simulink model "Kal_pitch_sim"  (R2023b)
settings: Solver=FixedStepAuto  StartTime=0.0  StopTime=50  FixedStep=0.001  RelTol=1e-3
values from neighbouring files (symbols this model uses):
  beta = pi/10    (= 0.314159265359)    [Kal_6Dpitch_mat.m]    (also in Kal_pitch_mat.m; TestValori.m = 0.523598775598; TestVel.m = 0.523598775598)
  cov_ic = [10, 0 ... (first row only)    [KalPrep_mat.m]    (also in Kal_6Dpitch_mat.m = cov_ic * (1 + 2*rand); Kal_pitch_mat.m = cov_ic * (1 + 2*rand))
  eta1 = deg2rad(1)    [KalPrep_mat.m]    (also in Kal_6Dpitch_mat.m = 0.05; Kal_pitch_mat.m = 0.05)
  eta2 = 0.05    [Kal_6Dpitch_mat.m]    (also in Kal_pitch_mat.m)
  G = [Ts 0 ... (first row only)    [KalPrep_mat.m]    (also in Kal_6Dpitch_mat.m = eye(3) * Ts; Kal_pitch_mat.m = eye(3) * Ts)
  Gamma = -pi/6    (= -0.523598775598)    [Kal_6Dpitch_mat.m]    (also in Kal_pitch_mat.m; TestValori.m)
  init_cond = [pi/2; 5]    [KalPrep_mat.m]    (also in Kal_6Dpitch_mat.m = [2; 0; 0]; Kal_pitch_mat.m = [2; 0; 0])
  Lambda = pi/6    (= 0.523598775598)    [Kal_6Dpitch_mat.m]    (also in Kal_pitch_mat.m; TestValori.m)
  pr0 = [0,0]'    [Kal_6Dpitch_mat.m]    (also in Kal_pitch_mat.m)
  Q = [(sig1^2), 0 ... (first row only)    [KalPrep_mat.m]    (also in Kal_6Dpitch_mat.m = zeros(3,3); Kal_pitch_mat.m = zeros(3,3))
  qt = - 10    (= -10)    [Kal_6Dpitch_mat.m]    (also in Kal_pitch_mat.m; TestValori.m = -5)
  R = (eta1)^2    [KalPrep_mat.m]    (also in Kal_6Dpitch_mat.m = [(eta1^2), 0; Kal_pitch_mat.m = [(eta1^2), 0; untitled.m = 10)
  sig1 = 0.1    [KalPrep_mat.m]    (also in Kal_6Dpitch_mat.m; Kal_pitch_mat.m)
  sig2 = 0.2    [KalPrep_mat.m]    (also in Kal_6Dpitch_mat.m; Kal_pitch_mat.m)
  sig3 = 0.15    [Kal_6Dpitch_mat.m]    (also in Kal_pitch_mat.m)
  Ts = 0.001    [KalPrep_mat.m]    (also in Kal_6Dpitch_mat.m; Kal_pitch_mat.m; TestVel.m)
  v_heave = 0.00    (= 0)    [Kal_pitch_mat.m]
  v_surge = 0.5    [Kal_pitch_mat.m]
settings Model: Creator=fabio  LastModifiedBy=fabio

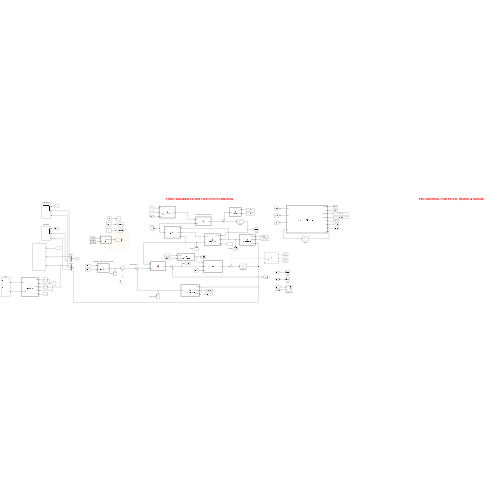
[thumbnail: Simulink's stored preview of the top-level diagram]
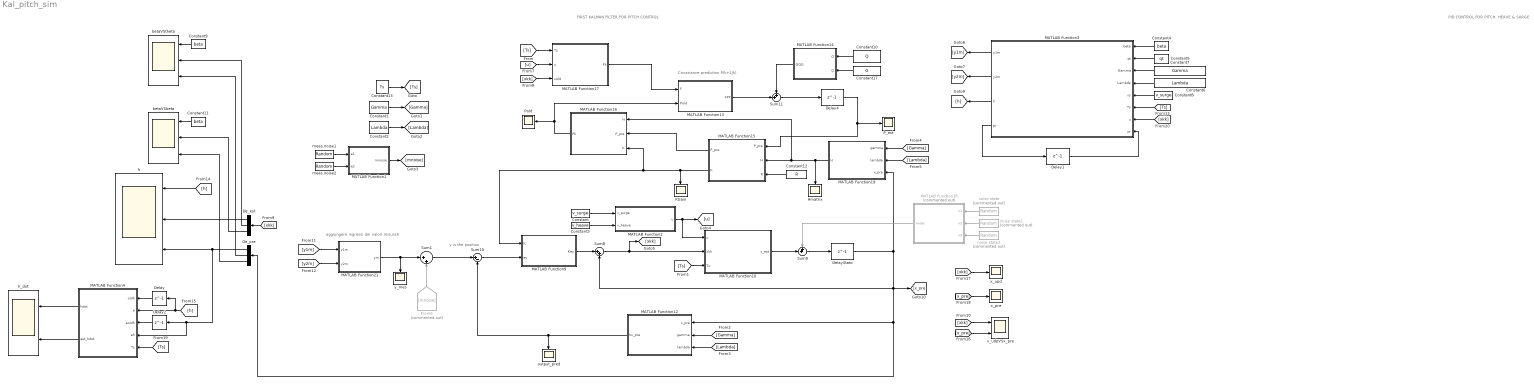
== system Kal_pitch_sim ==
  note: aggiungere ingressi dei valorì misurati
  note: Covariance prediction P(k+1|k)
  note: FIRST KALMAN FILTER FOR PITCH CONTROL
  note: y is the position
  note: PID CONTROL FOR PITCH, HEAVE & SURGE
  Constant : Constant  Value=v_surge
  Constant1 : Constant  Value=Gamma
  Constant10 : Constant  Value=Q  VectorParams1D=off
  Constant11 : Constant  Value=beta
  Constant12 : Constant  Value=R
  Constant13 : Constant  Value=Ts
  Constant17 : Constant  Value=G  VectorParams1D=off
  Constant2 : Constant  Value=Lambda
  Constant3 : Constant  Value=v_heave
  Constant4 : Constant  Value=beta
  Constant5 : Constant  Value=qt
  Constant6 : Constant  Value=Lambda
  Constant7 : Constant  Value=Gamma
  Constant8 : Constant  Value=v_surge
  Constant9 : Constant  Value=beta
  De_est : Demux  Outputs=3
  De_pre : Demux  Outputs=3
  Delay : Delay  DelayLength=1
  Delay1 : Delay  DelayLength=1  InitialCondition=pr0  UseCircularBuffer=on
  Delay2 : Delay  DelayLength=1
  Delay4 : Delay  DelayLength=1  InitialCondition=cov_ic  UseCircularBuffer=on
  DelayStato : Delay  DelayLength=1  InitialCondition=init_cond  UseCircularBuffer=on
  From6 : From  Commented=on  GotoTag=mnoise
  Hmatrix : Scope
  KGain : Scope
  MATLAB Function1 : MATLAB Function  TreatAsAtomicUnit=on
  MATLAB Function10 : MATLAB Function  TreatAsAtomicUnit=on
  MATLAB Function12 : MATLAB Function  TreatAsAtomicUnit=on
  MATLAB Function13 : MATLAB Function  TreatAsAtomicUnit=on
  MATLAB Function14 : MATLAB Function  TreatAsAtomicUnit=on
  MATLAB Function15 : MATLAB Function  TreatAsAtomicUnit=on
  MATLAB Function16 : MATLAB Function  TreatAsAtomicUnit=on
  MATLAB Function17 : MATLAB Function  TreatAsAtomicUnit=on
  MATLAB Function18 : MATLAB Function  Commented=on  TreatAsAtomicUnit=on
  MATLAB Function19 : MATLAB Function  TreatAsAtomicUnit=on
  MATLAB Function2 : MATLAB Function  TreatAsAtomicUnit=on
  MATLAB Function21 : MATLAB Function  TreatAsAtomicUnit=on
  MATLAB Function3 : MATLAB Function  TreatAsAtomicUnit=on
  MATLAB Function4 : MATLAB Function  TreatAsAtomicUnit=on
  MATLAB Function9 : MATLAB Function  TreatAsAtomicUnit=on
  P_est : Scope
  Pold : Scope
  Sum1 : Sum  Inputs=|++
  Sum10 : Sum  Inputs=|+-
  Sum11 : Sum  Inputs=++|
  Sum8 : Sum  Inputs=|++
  Sum9 : Sum  Inputs=++|
  betaVSbeta : Scope  NumInputPorts=3
  betaVStheta : Scope  NumInputPorts=3
  h : Scope  NumInputPorts=3
  h_dot : Scope  NumInputPorts=2
  meas.noise1 : RandomNumber  Variance=eta1  SampleTime=Ts
  meas.noise2 : RandomNumber  Variance=eta2  SampleTime=Ts
  noise state : RandomNumber  Commented=on  Variance=sig1  SampleTime=Ts
  noise state1 : RandomNumber  Commented=on  Variance=sig2  SampleTime=Ts
  noise state2 : RandomNumber  Commented=on  Variance=sig3  SampleTime=Ts
  output_pred : Scope
  x_pre : Scope
  x_udpVSx_pre : Scope  NumInputPorts=2
  x_upd : Scope
  y_mes : Scope
  wires:
  MATLAB Function17/1(Fk) -> MATLAB Function13/1(F)
  DelayStato/1 -> Sum8/2, [x_pre], MATLAB Function12/1(x_pre), De_pre/1, MATLAB Function19/3(x_pre)
  Delay4/1 -> P_est/1, MATLAB Function15/1("P_pre ")
  MATLAB Function12/1(hx_pre) -> Sum10/2, output_pred/1
  Sum10/1 -> MATLAB Function9/2(ey)
  MATLAB Function19/1(H) -> Hmatrix/1, MATLAB Function16/1(H), MATLAB Function15/2(H)
  Constant17/1 -> MATLAB Function14/2(G)
  MATLAB Function14/1(GQG) -> Sum11/1
  MATLAB Function13/1(FPF) -> Sum11/2
  Constant10/1 -> MATLAB Function14/1(Q)
  MATLAB Function10/1(x_est) -> Sum9/2
  MATLAB Function16/1(Pk) -> Pold/1, MATLAB Function13/2(Pold)
  Sum9/1 -> DelayStato/1
  Constant12/1 -> MATLAB Function15/3(R)
  MATLAB Function15/2(K) -> KGain/1, MATLAB Function16/3(K), MATLAB Function9/1(K)
  Sum11/1 -> Delay4/1
  Sum8/1 -> [xkk], MATLAB Function10/2(xkk)
  MATLAB Function15/1(P_pre) -> MATLAB Function16/2(P_pre)
  MATLAB Function9/1(Key) -> Sum8/1
  MATLAB Function21/1(ym) -> y_mes/1, Sum1/1
  Constant13/1 -> [Ts]
  [Ts] -> MATLAB Function17/1(Ts)
  [Ts] -> MATLAB Function10/3(Ts)
  Constant1/1 -> [Gamma]
  Constant2/1 -> [Lambda]
  [Gamma] -> MATLAB Function12/2(gamma)
  [Lambda] -> MATLAB Function12/3(lambda)
  [Gamma] -> MATLAB Function19/1(gamma)
  [Lambda] -> MATLAB Function19/2(lambda)
  noise state/1 -> MATLAB Function18/1(n1)
  noise state2/1 -> MATLAB Function18/3(n3)
  noise state1/1 -> MATLAB Function18/2(n2)
  MATLAB Function18/1(noise) -> Sum9/1
  Sum1/1 -> Sum10/1
  meas.noise1/1 -> MATLAB Function1/1(e1)
  meas.noise2/1 -> MATLAB Function1/2(e2)
  MATLAB Function1/1(mnoise) -> [mnoise]
  Constant/1 -> MATLAB Function2/1(v_surge)
  MATLAB Function2/1(u) -> MATLAB Function10/1(u), [u]
  [u] -> MATLAB Function17/2(u)
  [xkk] -> MATLAB Function17/3(xold)
  Delay1/1 -> MATLAB Function3/8("pr ")
  MATLAB Function3/4(pr) -> Delay1/1
  MATLAB Function3/1(y1m) -> [y1m]
  MATLAB Function3/2(y2m) -> [y2m]
  [y1m] -> MATLAB Function21/1(y1m)
  [y2m] -> MATLAB Function21/2(y2m)
  Constant4/1 -> MATLAB Function3/1(beta)
  Constant5/1 -> MATLAB Function3/2(qt)
  Constant6/1 -> MATLAB Function3/4(Lambda)
  Constant8/1 -> MATLAB Function3/5(vs)
  [Ts] -> MATLAB Function3/6(Ts)
  MATLAB Function3/3(h) -> [h]
  [h] -> h/1
  [xkk] -> De_est/1
  De_est/1 -> h/2
  De_pre/1 -> MATLAB Function4/4(eh), Delay2/1, h/3
  Constant9/1 -> betaVStheta/1
  Constant7/1 -> MATLAB Function3/3(Gamma)
  MATLAB Function4/1(hdot) -> h_dot/1
  De_est/2 -> betaVStheta/2
  De_pre/2 -> betaVStheta/3
  De_est/3 -> betaVSbeta/2
  De_pre/3 -> betaVSbeta/3
  Constant11/1 -> betaVSbeta/1
  Constant3/1 -> MATLAB Function2/2(v_heave)
  [xkk] -> x_udpVSx_pre/1
  [x_pre] -> x_udpVSx_pre/2
  [xkk] -> x_upd/1
  [x_pre] -> x_pre/1
  MATLAB Function4/2(est_hdot) -> h_dot/2
  [h] -> Delay/1, MATLAB Function4/2(h)
  Delay/1 -> MATLAB Function4/1(oldh)
  Delay2/1 -> MATLAB Function4/3(eoldh)
  [Ts] -> MATLAB Function4/5(Ts)
  [xkk] -> MATLAB Function3/7(x)
  From6/1 -> Sum1/2

== matlab function Kal_pitch_sim/MATLAB Function16 ==
  data: H input; P_pre input; Pk output; K input
function Pk = PkComp(H ,P_pre, K)
    s = size((K*H), 1);
    I = eye(s); 
    Pk = (I - K*H)*P_pre;

== matlab function Kal_pitch_sim/MATLAB Function9 ==
  data: K input; ey input; Key output
function Key = GainMult(K, ey)
    Key = K*ey;

== matlab function Kal_pitch_sim/MATLAB Function17 ==
  data: Fk output; Ts input; u input; xold input
function Fk = DynamicJacobian(Ts, u, xold)
    delta = xold(3) - xold(2);
    % u(1) = vsurge, u(2) = vheave
    % !! ATTENZIONE:
    % STO CONSIDERANDO H RISPETTO TERRAIN FRAME E THETA E BETA RISPETTO
    % INERZIALE
    F = [0, -u(1)*cos(delta)+u(2)*sin(delta), u(1)*cos(delta)-u(2)*sin(delta);
            0, 0, 0;
            0, 0, 0];
    Fk = eye(3) + Ts * F;

== matlab function Kal_pitch_sim/MATLAB Function18 ==
  data: n1 input; n2 input; noise output; n3 input
function noise = StateNoise (n1, n2, n3)
    noise = [n1, n2, n3]';

== matlab function Kal_pitch_sim/MATLAB Function19 ==
  data: gamma input; lambda input; x_pre input; H output
function H = HComputation(gamma, lambda, x_pre)
    % x(1) = h, x(2) = theta, x(3) = beta
    % !! ATTENZIONE:
    % VA MODIFICATO E MESSO CON VALORE ASSOLUTO??
    delta = [(gamma - (x_pre(3) - x_pre(2)));
             (lambda - (x_pre(3) - x_pre(2)))];

    val1 = ((x_pre(1)*sin(delta(1))) / ((cos(delta(1)))^2));
    val2 = ((x_pre(1)*sin(delta(2))) / ((cos(delta(2)))^2)) * sign(cos(delta(1)));

    H = [(1/abs(cos(delta(1)))), val1 * sign(cos(delta(1))), -val1 * sign(cos(delta(1)));
         (1/abs(cos(delta(2)))), val2 * sign(cos(delta(2))), -val2 * sign(cos(delta(2)))];

== matlab function Kal_pitch_sim/MATLAB Function21 ==
  data: y1m input; y2m input; ym output
function ym = Ymeasured(y1m, y2m) 
    ym = [y1m; y2m];

== matlab function Kal_pitch_sim/MATLAB Function1 ==
  data: e1 input; e2 input; mnoise output
function mnoise = StateNoise (e1, e2)
    mnoise = [e1, e2]';

== matlab function Kal_pitch_sim/MATLAB Function2 ==
  data: v_surge input; v_heave input; u output
function u = InputCreation(v_surge, v_heave)
    u = [v_surge;
         v_heave];

== matlab function Kal_pitch_sim/MATLAB Function3 ==
  data: beta input; qt input; y1m output; Gamma input; Lambda input; vs input; Ts input; x input; y2m output; h output; pr input; pr output
function [y1m, y2m, h, pr] = MeasuramentComputation(beta, qt, Gamma, Lambda, vs, Ts, x, pr) 
    % terrain construction
    mt = tan(beta);
    m1_g = tan((3*pi/2 + Gamma + x(2)));  
    m2_l = tan((3*pi/2 + Lambda + x(2)));
    % robot position
    % pr(2) = 0 constant 
    pr(1) = pr(1) + Ts * vs;
    q1 = pr(2) - m1_g*pr(1);
    q2 = pr(2) - m2_l*pr(1);

    % computation for y1
    xc1 = (q1 - qt) / (mt - m1_g);
    yc1 = mt * xc1 + qt;
    y1m = norm([pr(1) - xc1; pr(2) - yc1]);

    % Computation for y2
    xc2 = (q2 - qt) / (mt - m2_l);
    yc2 = mt * xc2 + qt;
    y2m = norm([pr(1) - xc2; pr(2) - yc2]);
    
    % valore da ottenere di h
    h = (abs(mt*pr(1) - pr(2) + qt))/ (sqrt(mt^2 + 1));
end

== matlab function Kal_pitch_sim/MATLAB Function4 ==
  data: oldh input; h input; hdot output; eoldh input; eh input; Ts input; est_hdot output
function [hdot, est_hdot] =  Derivation(oldh, h, eoldh, eh, Ts)
    hdot = (h - oldh) / Ts;
    est_hdot = (eh - eoldh) / Ts;

== matlab function Kal_pitch_sim/MATLAB Function10 ==
  data: u input; xkk input; x_est output; Ts input
function x_est = StatePrediction(u, xkk, Ts)
    % xkk(3) = beta, xkk(2) = theta
    % u(1) = vsurge, u(2) = vheave
    A = eye(3);
    delta = xkk(3) - xkk(2);
    B = [-sin(delta), -cos(delta);
         0, 0;
         0, 0];
    x_est = A*xkk + B*u*Ts;

== matlab function Kal_pitch_sim/MATLAB Function12 ==
  data: x_pre input; hx_pre output; gamma input; lambda input
function hx_pre = OutputPrediction(x_pre, gamma, lambda)
    delta = [(gamma - (x_pre(3) - x_pre(2)));
             (lambda - (x_pre(3) - x_pre(2)))];
    
    hx_pre = [x_pre(1)/abs((cos(delta(1))));
              x_pre(1)/abs((cos(delta(2))))];

== matlab function Kal_pitch_sim/MATLAB Function13 ==
  data: F input; Pold input; FPF output
function FPF = FPFmatrix(F ,Pold)
    FPF = F*Pold*(F');

== matlab function Kal_pitch_sim/MATLAB Function14 ==
  data: Q input; GQG output; G input
function GQG = GmatrixQ(Q, G)
    GQG = G*Q*(G');

== matlab function Kal_pitch_sim/MATLAB Function15 ==
  data: P_pre output; P_pre input; H input; K output; R input
function [P_pre, K] = KalmanGain(P_pre, H, R)
    K = (P_pre*(H'))*pinv((H*P_pre*(H') + R)); 
    K(2,:) = 0; % non sto ancora curando theta
